simulink model "FiveStateAbsTcs"  (R2026b)
undefined symbols (not defined in the file): CtrlBcuTrlrBrkGain, CtrlTrgtWhlSlip, DiscIntNeverNeededParam, PlntVehInitLongVel, PlntWhlLdRadiusFrnt, PlntWhlLdRadiusRear
libraries: autolibsharedabs x1, simulink x1
settings Model: Creator=The MathWorks, Inc.  LastModifiedBy=The MathWorks, Inc.

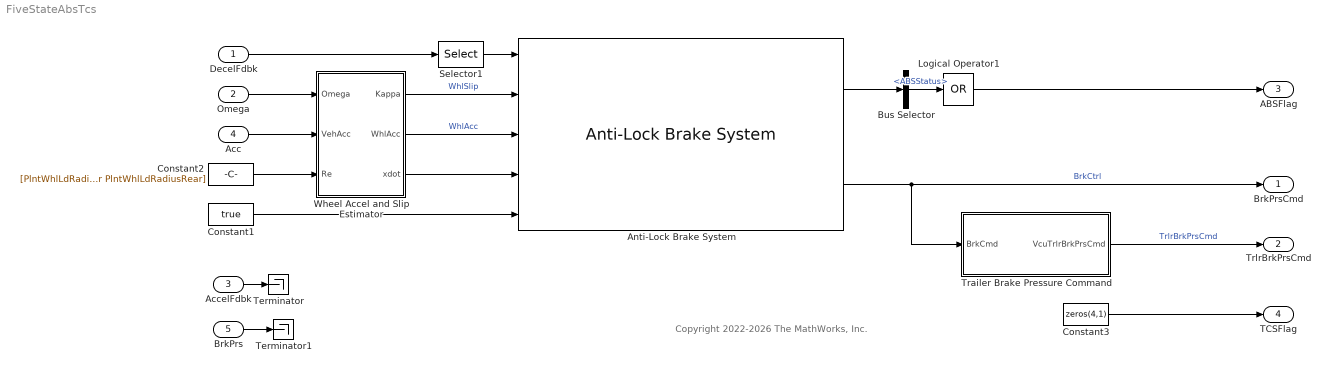
== system FiveStateAbsTcs ==
  note: Copyright 2022-2026 The MathWorks, Inc.
  DecelFdbk : Inport  OutDataTypeStr=double  PortDimensions=1
  Omega : Inport  Port=2  OutDataTypeStr=double  PortDimensions=4
  AccelFdbk : Inport  Port=3  OutDataTypeStr=double  PortDimensions=1
  Acc : Inport  Port=4  OutDataTypeStr=double  PortDimensions=1
  BrkPrs : Inport  Port=5  OutDataTypeStr=double  PortDimensions=4
  Anti-Lock Brake System : autolibsharedabs/Anti-Lock Brake System  VariantControl=Three Axle Trailer ABS Control Felix  TrgtWhlSlip=CtrlTrgtWhlSlip*ones(1,4)  AbsEnBrkThr=0.05*ones(1,4)  AbsEnSpdThr=1  Unit=m/s  InitBrkCmd=0  BrkReleaseRate=-5*ones(1,4)  BrkHldRate=0  BrkMildIncRate=10*ones(1,4)  BrkRapidIncRate=20*ones(1,4)  AccelLowrLmt=2*ones(1,4)  AccelUpprLmt=100*ones(1,4)  HdOffTime=0.2  BrkCtrlLmt=0.01*ones(1,4)  aMode=2
      settings: LibrarySourceBlock=vehdynlibcontrol/Anti-Lock Brake System
  Bus Selector : BusSelector  OutputSignals=ABSStatus
  Constant1 : Constant  Value=true  SampleTime=-1
  Constant2 : Constant  Value=[PlntWhlLdRadiusFrnt PlntWhlLdRadiusFrnt PlntWhlLdRadiusRear PlntWhlLdRadiusRear]  SampleTime=-1
  Constant3 : Constant  Value=zeros(4,1)  SampleTime=-1
  Logical Operator1 : Logic  Operator=OR  Inputs=1  AllPortsSameDT=off  OutDataTypeStr=boolean
  Selector1 : Selector  InputPortWidth=1  IndexOptions=Index vector (dialog)  Indices=[1 1 1 1]  OutputSizes=1
  Terminator : Terminator
  Terminator1 : Terminator
  Trailer Brake Pressure Command : Subsystem
  Wheel Accel and Slip Estimator : Subsystem
  BrkPrsCmd : Outport  OutDataTypeStr=double  PortDimensions=4
  TrlrBrkPrsCmd : Outport  Port=2  PortDimensions=6  VectorParamsAs1DForOutWhenUnconnected=off
  ABSFlag : Outport  Port=3
  TCSFlag : Outport  Port=4  OutDataTypeStr=double  PortDimensions=4
  wires:
  Anti-Lock Brake System/2 -> BrkPrsCmd/1, Trailer Brake Pressure Command/1(BrkCmd)  "BrkCtrl"
  Wheel Accel and Slip Estimator/2(WhlAcc) -> Anti-Lock Brake System/3  "WhlAcc"
  Wheel Accel and Slip Estimator/1(Kappa) -> Anti-Lock Brake System/2  "WhlSlip"
  Omega/1 -> Wheel Accel and Slip Estimator/1(Omega)
  Acc/1 -> Wheel Accel and Slip Estimator/2(VehAcc)
  Logical Operator1/1 -> ABSFlag/1
  Trailer Brake Pressure Command/1(VcuTrlrBrkPrsCmd) -> TrlrBrkPrsCmd/1  "TrlrBrkPrsCmd"
  Constant1/1 -> Anti-Lock Brake System/5
  Constant2/1 -> Wheel Accel and Slip Estimator/3(Re)
  DecelFdbk/1 -> Selector1/1
  Wheel Accel and Slip Estimator/3(xdot) -> Anti-Lock Brake System/4
  Selector1/1 -> Anti-Lock Brake System/1
  AccelFdbk/1 -> Terminator/1
  BrkPrs/1 -> Terminator1/1
  Constant3/1 -> TCSFlag/1
  Anti-Lock Brake System/1 -> Bus Selector/1
  Bus Selector/1 -> Logical Operator1/1  "<ABSStatus>"

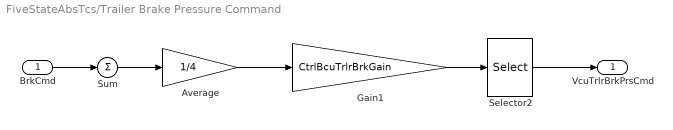
== system FiveStateAbsTcs/Trailer Brake Pressure Command ==
  BrkCmd : Inport
  Average : Gain  Gain=1/4
  Gain1 : Gain  Gain=CtrlBcuTrlrBrkGain
  Selector2 : Selector  InputPortWidth=1  IndexOptions=Index vector (dialog)  Indices=[1 1 1 1 1 1]  OutputSizes=1
  Sum : Sum  Inputs=+
  VcuTrlrBrkPrsCmd : Outport
  wires:
  Gain1/1 -> Selector2/1
  Average/1 -> Gain1/1
  BrkCmd/1 -> Sum/1
  Sum/1 -> Average/1
  Selector2/1 -> VcuTrlrBrkPrsCmd/1

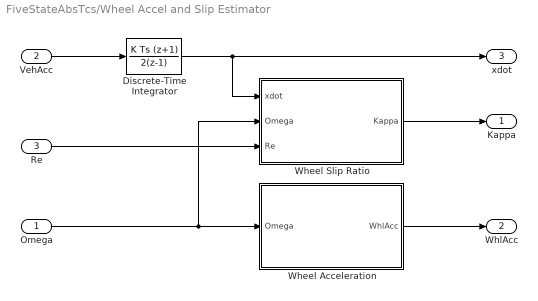
== system FiveStateAbsTcs/Wheel Accel and Slip Estimator ==
  Omega : Inport
  VehAcc : Inport  Port=2
  Re : Inport  Port=3
  Discrete-Time Integrator : DiscreteIntegrator  IntegratorMethod=Integration: Trapezoidal  InitialCondition=PlntVehInitLongVel  SampleTime=-1  ICPrevOutput=DiscIntNeverNeededParam  ICPrevScaledInput=DiscIntNeverNeededParam
  Wheel Acceleration : Subsystem  TreatAsAtomicUnit=on
  Wheel Slip Ratio : Subsystem  TreatAsAtomicUnit=on
  Kappa : Outport
  WhlAcc : Outport  Port=2  Unit=rad/s^2
  xdot : Outport  Port=3  Unit=m/s
  wires:
  Discrete-Time Integrator/1 -> xdot/1, Wheel Slip Ratio/1(xdot)
  VehAcc/1 -> Discrete-Time Integrator/1
  Omega/1 -> Wheel Slip Ratio/2(Omega), Wheel Acceleration/1(Omega)
  Wheel Acceleration/1(WhlAcc) -> WhlAcc/1
  Wheel Slip Ratio/1(Kappa) -> Kappa/1
  Re/1 -> Wheel Slip Ratio/3(Re)

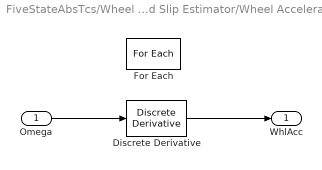
== system FiveStateAbsTcs/Wheel Accel and Slip Estimator/Wheel Acceleration ==
  Omega : Inport  PortDimensions=1  Partition=on  PartitionDimension=1  PartitionWidth=1  PartitionOffset=0
  Discrete Derivative : simulink/Discrete/Discrete Derivative  gainval=1.0  ICPrevScaledInput=0.0  OutMin=[]  OutMax=[]  OutDataType=fixdt(1, 16)  OutScaling=2^-10  DoSatur=off
  For Each : ForEach  DisableCoverage=on
  WhlAcc : Outport  ConcatenationDimension=1
  wires:
  Omega/1 -> Discrete Derivative/1
  Discrete Derivative/1 -> WhlAcc/1

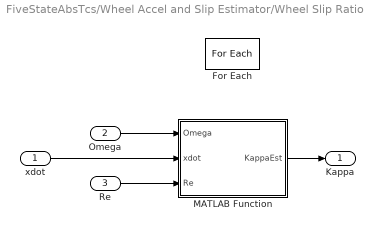
== system FiveStateAbsTcs/Wheel Accel and Slip Estimator/Wheel Slip Ratio ==
  xdot : Inport
  Omega : Inport  Port=2  PortDimensions=1  Partition=on  PartitionDimension=1  PartitionWidth=1  PartitionOffset=0
  Re : Inport  Port=3  PortDimensions=1  Partition=on  PartitionDimension=1  PartitionWidth=1  PartitionOffset=0
  For Each : ForEach  DisableCoverage=on
  MATLAB Function : MATLAB Function  TreatAsAtomicUnit=on
  Kappa : Outport  ConcatenationDimension=1
  wires:
  MATLAB Function/1(KappaEst) -> Kappa/1
  xdot/1 -> MATLAB Function/2(xdot)
  Omega/1 -> MATLAB Function/1(Omega)
  Re/1 -> MATLAB Function/3(Re)

== matlab function FiveStateAbsTcs/Wheel Accel and Slip Estimator/Wheel Slip Ratio/MATLAB Function ==
  data: Omega input; xdot input; KappaEst output; Re input
function KappaEst = fcn(Omega, xdot, Re)

WhlSpd = Omega * Re;

if WhlSpd ~= 0 || xdot ~= 0
    KappaEst = (WhlSpd - xdot) / max([abs(xdot) abs(WhlSpd)]);
else
    KappaEst = 0;
end
